simulink library "Magnetometer"  (R2014b)
settings: Solver=VariableStepAuto  StartTime=0.0  StopTime=10.0  RelTol=1e-3
undefined symbols (not defined in the file or in its folder): ConfParam
libraries: simulink x1, ChangeFrame x1
settings Model: Creator=y.akisheva  LastModifiedBy=Hp
settings DataIOCC: SaveFormat=Dataset
settings OptimizationCC: UseDivisionForNetSlopeComputation=off  SimCompilerOptimization=off
settings DebuggingCC: SolverPrmCheckMsg=none  FrameProcessingCompatibilityMsg=error  AllowSymbolicDim=off
settings HardwareCC: ProdBitPerPointer=64  ProdLargestAtomicFloat=Float  ProdIntDivRoundTo=Zero  ProdEndianess=LittleEndian  ProdWordSize=64  ProdHWDeviceType=Intel->x86-64 (Windows64)
settings RTWCC: RTWCompilerOptimization=off
settings GRTTargetCC: GeneratePreprocessorConditionals=Use local settings
settings ConfigComp: CovMetricSettings=dw  CovHtmlReporting=on  CovSaveCumulativeToWorkspaceVar=on  CovSaveSingleToWorkspaceVar=on  CovExternalEMLEnable=off

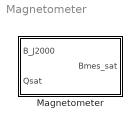
== system Magnetometer ==
  Magnetometer : Subsystem

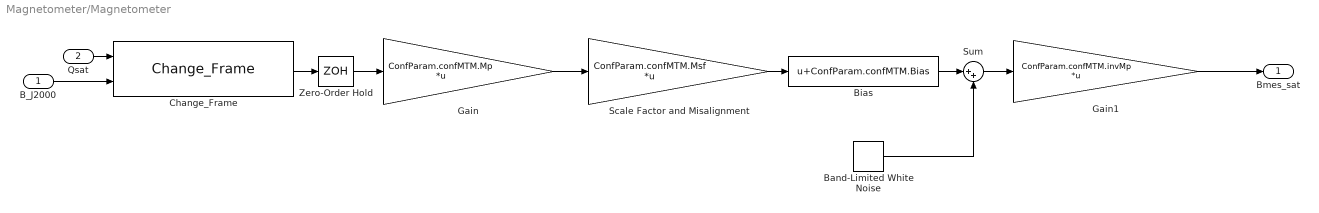
== system Magnetometer/Magnetometer ==
  B_J2000 : Inport
  Qsat : Inport  Port=2
  Band-Limited White Noise : simulink/Sources/Band-Limited White Noise  Cov=ConfParam.confMTM.NoisePower  Ts=1/ConfParam.confMTM.frequency  seed=[23341]
  Bias : Bias  Bias=ConfParam.confMTM.Bias
  Change_Frame : ChangeFrame/Change_Frame
  Gain : Gain  Gain=ConfParam.confMTM.Mp  Multiplication=Matrix(K*u)
  Gain1 : Gain  Gain=ConfParam.confMTM.invMp  Multiplication=Matrix(K*u)
  Scale Factor and Misalignment : Gain  Gain=ConfParam.confMTM.Msf  Multiplication=Matrix(K*u)
  Sum : Sum  Inputs=|++
  Zero-Order Hold : ZeroOrderHold  SampleTime=1/ConfParam.confMTM.frequency
  Bmes_sat : Outport
  wires:
  Bias/1 -> Sum/1
  Sum/1 -> Gain1/1
  B_J2000/1 -> Change_Frame/2
  Scale Factor and Misalignment/1 -> Bias/1
  Band-Limited White Noise/1 -> Sum/2
  Gain/1 -> Scale Factor and Misalignment/1
  Gain1/1 -> Bmes_sat/1
  Zero-Order Hold/1 -> Gain/1
  Change_Frame/1 -> Zero-Order Hold/1
  Qsat/1 -> Change_Frame/1
